simulink model "amr_scenario_supervisor"  (R2025b)
settings: Solver=FixedStepDiscrete  StartTime=0.0  StopTime=90  FixedStep=0.05  RelTol=1e-3
settings Model: Creator=leeyj  LastModifiedBy=leeyj

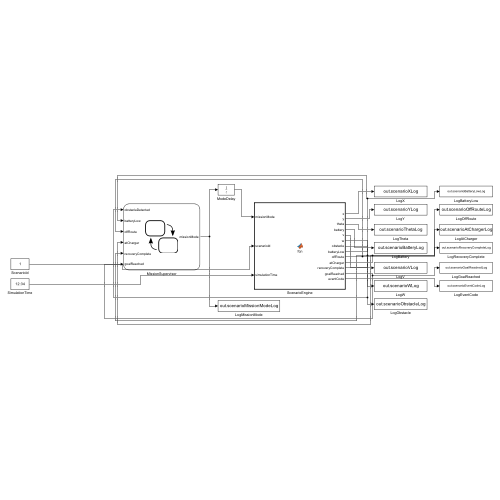
[thumbnail: Simulink's stored preview of the top-level diagram]
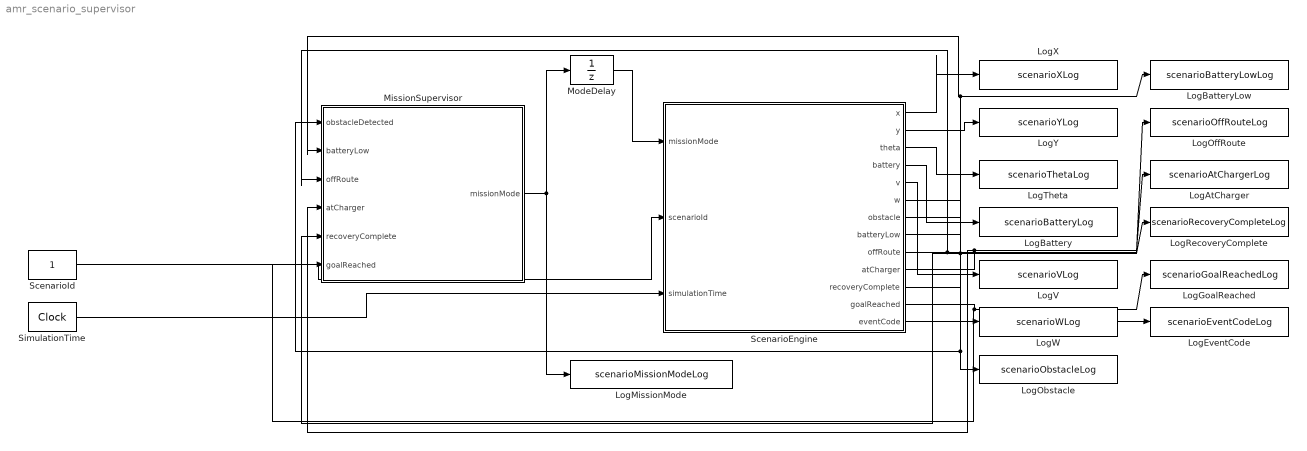
== system amr_scenario_supervisor ==
  LogAtCharger : ToWorkspace  VariableName=scenarioAtChargerLog  SaveFormat=Timeseries  SampleTime=-1
  LogBattery : ToWorkspace  VariableName=scenarioBatteryLog  SaveFormat=Timeseries  SampleTime=-1
  LogBatteryLow : ToWorkspace  VariableName=scenarioBatteryLowLog  SaveFormat=Timeseries  SampleTime=-1
  LogEventCode : ToWorkspace  VariableName=scenarioEventCodeLog  SaveFormat=Timeseries  SampleTime=-1
  LogGoalReached : ToWorkspace  VariableName=scenarioGoalReachedLog  SaveFormat=Timeseries  SampleTime=-1
  LogMissionMode : ToWorkspace  VariableName=scenarioMissionModeLog  SaveFormat=Timeseries  SampleTime=-1
  LogObstacle : ToWorkspace  VariableName=scenarioObstacleLog  SaveFormat=Timeseries  SampleTime=-1
  LogOffRoute : ToWorkspace  VariableName=scenarioOffRouteLog  SaveFormat=Timeseries  SampleTime=-1
  LogRecoveryComplete : ToWorkspace  VariableName=scenarioRecoveryCompleteLog  SaveFormat=Timeseries  SampleTime=-1
  LogTheta : ToWorkspace  VariableName=scenarioThetaLog  SaveFormat=Timeseries  SampleTime=-1
  LogV : ToWorkspace  VariableName=scenarioVLog  SaveFormat=Timeseries  SampleTime=-1
  LogW : ToWorkspace  VariableName=scenarioWLog  SaveFormat=Timeseries  SampleTime=-1
  LogX : ToWorkspace  VariableName=scenarioXLog  SaveFormat=Timeseries  SampleTime=-1
  LogY : ToWorkspace  VariableName=scenarioYLog  SaveFormat=Timeseries  SampleTime=-1
  MissionSupervisor : Stateflow chart  TreatAsAtomicUnit=on
  ModeDelay : UnitDelay  SampleTime=0.05  HasFrameUpgradeWarning=on
  ScenarioEngine : MATLAB Function  TreatAsAtomicUnit=on
  ScenarioId : Constant
  SimulationTime : DigitalClock  SampleTime=0.05
  wires:
  ModeDelay/1 -> ScenarioEngine/1(missionMode)
  ScenarioId/1 -> ScenarioEngine/2(scenarioId)
  SimulationTime/1 -> ScenarioEngine/3(simulationTime)
  ScenarioEngine/1(x) -> LogX/1
  ScenarioEngine/2(y) -> LogY/1
  ScenarioEngine/3(theta) -> LogTheta/1
  ScenarioEngine/4(battery) -> LogBattery/1
  ScenarioEngine/5(v) -> LogV/1
  ScenarioEngine/6(w) -> LogW/1
  ScenarioEngine/7(obstacle) -> MissionSupervisor/1(obstacleDetected), LogObstacle/1
  ScenarioEngine/8(batteryLow) -> LogBatteryLow/1, MissionSupervisor/2(batteryLow)
  ScenarioEngine/9(offRoute) -> LogOffRoute/1, MissionSupervisor/3(offRoute)
  ScenarioEngine/10(atCharger) -> LogAtCharger/1, MissionSupervisor/4(atCharger)
  ScenarioEngine/11(recoveryComplete) -> LogRecoveryComplete/1, MissionSupervisor/5(recoveryComplete)
  ScenarioEngine/12(goalReached) -> LogGoalReached/1, MissionSupervisor/6(goalReached)
  ScenarioEngine/13(eventCode) -> LogEventCode/1
  MissionSupervisor/1(missionMode) -> ModeDelay/1, LogMissionMode/1

== matlab function amr_scenario_supervisor/ScenarioEngine ==
  data: x output double size=1; missionMode input uint8 size=1; y output double size=1; scenarioId input double size=1; simulationTime input double size=1; theta output double size=1; battery output double size=1; v output double size=1; w output double size=1; obstacle output boolean size=1; batteryLow output boolean size=1; offRoute output boolean size=1; atCharger output boolean size=1; recoveryComplete output boolean size=1; goalReached output boolean size=1; eventCode output uint8 size=1
function [x,y,theta,battery,v,w,obstacle,batteryLow,offRoute,atCharger,recoveryComplete,goalReached,eventCode] = fcn(missionMode,scenarioId,simulationTime)
coder.extrinsic('amr.scenarios.scenarioEngineStep');
x=0.0; y=0.0; theta=0.0; battery=0.0; v=0.0; w=0.0;
obstacle=false; batteryLow=false; offRoute=false; atCharger=false; recoveryComplete=false; goalReached=false; eventCode=uint8(0);
[x,y,theta,battery,v,w,obstacle,batteryLow,offRoute,atCharger,recoveryComplete,goalReached,eventCode] = amr.scenarios.scenarioEngineStep(uint8(missionMode),scenarioId,simulationTime);

== stateflow chart amr_scenario_supervisor/MissionSupervisor ==
  state Rerouting
    entry,during:
    missionMode = uint8(7);
  state OffRouteStop
    entry,during:
    missionMode = uint8(6);
  state Initializing
    entry,during:
    missionMode = uint8(0);
  state Completed
    entry,during:
    missionMode = uint8(8);
  state Charging
    entry,during:
    missionMode = uint8(5);
  state Delivering
    entry,during:
    missionMode = uint8(1);
  state ReturnToCharger
    entry,during:
    missionMode = uint8(4);
  state ObstacleStop
    entry,during:
    missionMode = uint8(2);
  state AvoidingObstacle
    entry,during:
    missionMode = uint8(3);
  (default) -> Initializing
  OffRouteStop -> Rerouting : after(1,sec)
  Rerouting -> Delivering : [recoveryComplete]
  Delivering -> OffRouteStop [order 3] : [offRoute]
  Initializing -> Delivering : after(1,sec)
  Delivering -> Completed [order 4] : [goalReached]
  Delivering -> ObstacleStop [order 1] : [obstacleDetected]
  Charging -> Delivering : [recoveryComplete]
  AvoidingObstacle -> Delivering : [recoveryComplete]
  Delivering -> ReturnToCharger [order 2] : [batteryLow]
  ReturnToCharger -> Charging : [atCharger]
  ObstacleStop -> AvoidingObstacle : after(1,sec)
  data: obstacleDetected input boolean; batteryLow input boolean; offRoute input boolean; atCharger input boolean; recoveryComplete input boolean; goalReached input boolean; missionMode output uint8
